simulink model "SNS_Deng_PF"  (R2025a)
settings: Solver=ode1  StartTime=0.0  StopTime=10.0  FixedStep=1e-4  RelTol=1e-3
libraries: SNS_Library x16, SNS_Deng_Library x4
settings Model: Creator=Ben Bolen  LastModifiedBy=Ben Bolen

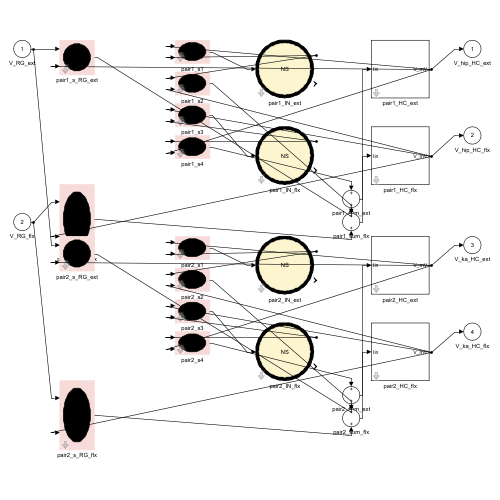
[thumbnail: Simulink's stored preview of the top-level diagram]
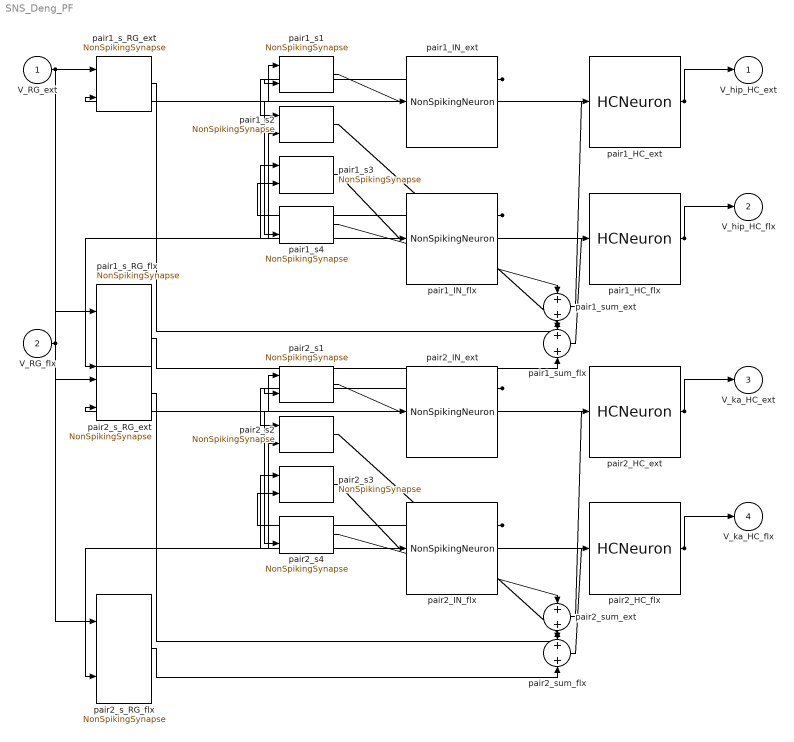
== system SNS_Deng_PF ==
  V_RG_ext : Inport
  V_RG_flx : Inport  Port=2
  pair1_HC_ext : SNS_Deng_Library/HCNeuron  Cm=5  Gm=1  Vrest=-60  GNa=1.5  ENa=50  Sm=0.2  Em=-40  Km=1  Sh=-0.6  Eh=-60  Kh=0.5  tauH=350  h0=0.6666667
  pair1_HC_flx : SNS_Deng_Library/HCNeuron  Cm=5  Gm=1  Vrest=-60  GNa=1.5  ENa=50  Sm=0.2  Em=-40  Km=1  Sh=-0.6  Eh=-60  Kh=0.5  tauH=350  h0=0.6666667
  pair1_IN_ext : SNS_Library/NonSpikingNeuron  Vrest=-60  Gm=1  Cm=5  Thr=-60  Slope=35
  pair1_IN_flx : SNS_Library/NonSpikingNeuron  Vrest=-60  Gm=1  Cm=5  Thr=-60  Slope=35
  pair1_s1 : SNS_Library/NonSpikingSynapse  gmax=2.749  Esyn=-40  ThrPre=-60  SlopePre=35
  pair1_s2 : SNS_Library/NonSpikingSynapse  gmax=2.749  Esyn=-70  ThrPre=-60  SlopePre=35
  pair1_s3 : SNS_Library/NonSpikingSynapse  gmax=2.749  Esyn=-40  ThrPre=-60  SlopePre=35
  pair1_s4 : SNS_Library/NonSpikingSynapse  gmax=2.749  Esyn=-70  ThrPre=-60  SlopePre=35
  pair1_s_RG_ext : SNS_Library/NonSpikingSynapse  gmax=0.1  Esyn=-40  ThrPre=-60  SlopePre=20
  pair1_s_RG_flx : SNS_Library/NonSpikingSynapse  gmax=0.1  Esyn=-40  ThrPre=-60  SlopePre=20
  pair1_sum_ext : Sum
  pair1_sum_flx : Sum
  pair2_HC_ext : SNS_Deng_Library/HCNeuron  Cm=5  Gm=1  Vrest=-60  GNa=1.5  ENa=50  Sm=0.2  Em=-40  Km=1  Sh=-0.6  Eh=-60  Kh=0.5  tauH=350  h0=0.6666667
  pair2_HC_flx : SNS_Deng_Library/HCNeuron  Cm=5  Gm=1  Vrest=-60  GNa=1.5  ENa=50  Sm=0.2  Em=-40  Km=1  Sh=-0.6  Eh=-60  Kh=0.5  tauH=350  h0=0.6666667
  pair2_IN_ext : SNS_Library/NonSpikingNeuron  Vrest=-60  Gm=1  Cm=5  Thr=-60  Slope=35
  pair2_IN_flx : SNS_Library/NonSpikingNeuron  Vrest=-60  Gm=1  Cm=5  Thr=-60  Slope=35
  pair2_s1 : SNS_Library/NonSpikingSynapse  gmax=2.749  Esyn=-40  ThrPre=-60  SlopePre=35
  pair2_s2 : SNS_Library/NonSpikingSynapse  gmax=2.749  Esyn=-70  ThrPre=-60  SlopePre=35
  pair2_s3 : SNS_Library/NonSpikingSynapse  gmax=2.749  Esyn=-40  ThrPre=-60  SlopePre=35
  pair2_s4 : SNS_Library/NonSpikingSynapse  gmax=2.749  Esyn=-70  ThrPre=-60  SlopePre=35
  pair2_s_RG_ext : SNS_Library/NonSpikingSynapse  gmax=0.1  Esyn=-40  ThrPre=-60  SlopePre=20
  pair2_s_RG_flx : SNS_Library/NonSpikingSynapse  gmax=0.1  Esyn=-40  ThrPre=-60  SlopePre=20
  pair2_sum_ext : Sum
  pair2_sum_flx : Sum
  V_hip_HC_ext : Outport
  V_hip_HC_flx : Outport  Port=2
  V_ka_HC_ext : Outport  Port=3
  V_ka_HC_flx : Outport  Port=4
  wires:
  pair1_HC_ext/1 -> pair1_s1/1, pair1_s4/2, pair1_s_RG_ext/2, V_hip_HC_ext/1
  pair1_IN_ext/1 -> pair1_s1/2, pair1_s2/1
  pair1_s1/1 -> pair1_IN_ext/1
  pair1_HC_flx/1 -> pair1_s2/2, pair1_s3/1, pair1_s_RG_flx/2, V_hip_HC_flx/1
  pair1_IN_flx/1 -> pair1_s3/2, pair1_s4/1
  pair1_s3/1 -> pair1_IN_flx/1
  pair1_s4/1 -> pair1_sum_ext/1
  pair1_s2/1 -> pair1_sum_flx/1
  pair1_sum_ext/1 -> pair1_HC_ext/1
  pair1_sum_flx/1 -> pair1_HC_flx/1
  V_RG_ext/1 -> pair1_s_RG_ext/1, pair2_s_RG_ext/1
  pair1_s_RG_ext/1 -> pair1_sum_ext/2
  V_RG_flx/1 -> pair1_s_RG_flx/1, pair2_s_RG_flx/1
  pair1_s_RG_flx/1 -> pair1_sum_flx/2
  pair2_HC_ext/1 -> pair2_s1/1, pair2_s4/2, pair2_s_RG_ext/2, V_ka_HC_ext/1
  pair2_IN_ext/1 -> pair2_s1/2, pair2_s2/1
  pair2_s1/1 -> pair2_IN_ext/1
  pair2_HC_flx/1 -> pair2_s2/2, pair2_s3/1, pair2_s_RG_flx/2, V_ka_HC_flx/1
  pair2_IN_flx/1 -> pair2_s3/2, pair2_s4/1
  pair2_s3/1 -> pair2_IN_flx/1
  pair2_s4/1 -> pair2_sum_ext/1
  pair2_s2/1 -> pair2_sum_flx/1
  pair2_sum_ext/1 -> pair2_HC_ext/1
  pair2_sum_flx/1 -> pair2_HC_flx/1
  pair2_s_RG_ext/1 -> pair2_sum_ext/2
  pair2_s_RG_flx/1 -> pair2_sum_flx/2
